simulink model "MdXX_StatusToNetWork"  (R2024b)
settings: Solver=FixedStepDiscrete  StartTime=0.0  StopTime=10.0  FixedStep=0.01  RelTol=1e-3
undefined symbols (not defined in the file or in its folder): KeSMSbSRSPosNumConfig_Val
(part 1 of 2)
settings Model: Creator=sn2xws  LastModifiedBy=sn55gm
settings Model: ModifiedHistory=|
  | 24.8.20 V3.0.0 557新增Md53 Md56
  | 24.10.15 V3.0.1 新增Md57 58
  | 25.7.4 V3.13.0 新增Md61 Md62
settings SolverCC: AlgebraicLoopSolver=TrustRegion
settings DataIOCC: SaveFormat=StructureWithTime  ReturnWorkspaceOutputs=off
settings OptimizationCC: DefaultParameterBehavior=Inlined  EnhancedBackFolding=on  PassReuseOutputArgsAs=Individual arguments  ZeroExternalMemoryAtStartup=off  ZeroInternalMemoryAtStartup=off  OptimizeBlockOrder=speed  DifferentSizesBufferReuse=on  OptimizationCustomize=off  EfficientTunableParamExpr=on
settings DebuggingCC: ParameterTunabilityLossMsg=error  UnconnectedInputMsg=warning  UnconnectedOutputMsg=warning  UnconnectedLineMsg=warning  ArithmeticOperatorsInVariantConditions=warning
settings ModelReferenceCC: EnableRefExpFcnMdlSchedulingChecks=on  ModelReferenceNumInstancesAllowed=Single
settings SFSimCC: MATLABDynamicMemAlloc=off  CustomCodeUndefinedFunction=UseInterfaceOnly
settings RTWCC: Description=AUTOSAR  SystemTargetFile=autosar.tlc  GenCodeOnly=on  TemplateMakefile=ert_default_tmf  GenerateReport=on  IncludeHyperlinkInReport=on  LaunchReport=on  DataTypeReplacement=CDataTypesFixedWidth  GenerateTraceInfo=on  GenerateTraceReport=on  GenerateTraceReportSl=on  GenerateTraceReportSf=on  GenerateTraceReportEml=on  GenerateCodeMetricsReport=on  GPUComputeCapability=3.5
settings CodeAppCC: ForceParamTrailComments=on  IgnoreCustomStorageClasses=off  OperatorAnnotations=on  SimulinkDataObjDesc=on  SFDataObjDesc=on  InsertBlockDesc=on
settings STFCustomTargetCC: TargetLangStandard=C99 (ISO)  MultiwordLength=256  ParMdlRefBuildCompliant=on  CompOptLevelCompliant=on  IncludeMdlTerminateFcn=off  CombineOutputUpdateFcns=on  SuppressErrorStatus=on  ERTCustomFileBanners=on  SupportNonFinite=off  SupportComplex=off  SupportContinuousTime=off  SupportNonInlinedSFcns=off  RemoveResetFunc=on  MATLABClassNameForMDSCustomization=Simulink.SoftwareTarget.ERTCustomization  AutosarCompliant=on  UseToolchainInfoCompliant=on  LookupTableObjectStructAxisOrder=2,1,3,4,...  LUTObjectStructOrderEvenSpacing=Size,Table,Breakpoints  SystemTargetFile=autosar.tlc
settings ERTTargetCC: TargetLangStandard=C99 (ISO)  ConcurrentExecutionCompliant=off  IncludeMdlTerminateFcn=off  SuppressErrorStatus=on  SupportNonFinite=off  SupportComplex=off  ModelStepFunctionPrototypeControlCompliant=off  CPPClassGenCompliant=off  AutosarCompliant=on  LookupTableObjectStructAxisOrder=2,1,3,4,...  LUTObjectStructOrderEvenSpacing=Size,Table,Breakpoints  ERTCustomFileTemplate=example_file_process.tlc  ERTFilePackagingFormat=Compact  BooleanTrueId=TRUE  BooleanFalseId=FALSE  DynamicArrayContainerType=coder::array

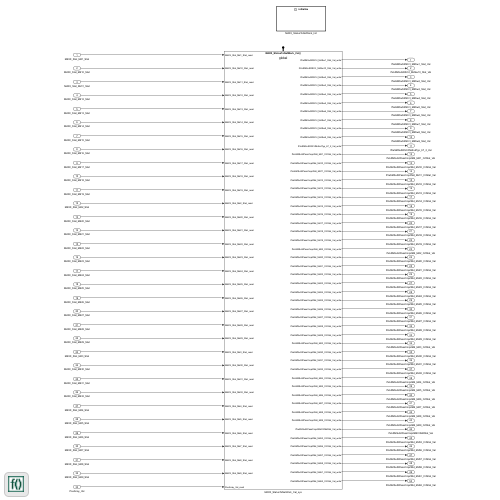
[thumbnail: Simulink's stored preview of the top-level diagram]
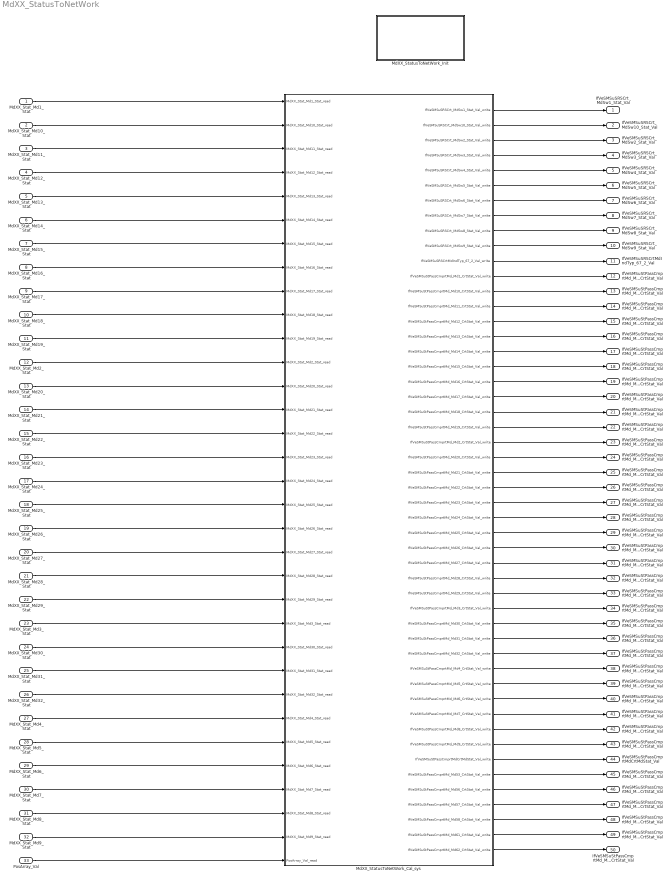
== system MdXX_StatusToNetWork ==
  MdXX_Stat_Md1_Stat : Inport  OutDataTypeStr=uint8  PortDimensions=1
  MdXX_Stat_Md10_Stat : Inport  Port=2  OutDataTypeStr=uint8  PortDimensions=1
  MdXX_Stat_Md11_Stat : Inport  Port=3  OutDataTypeStr=uint8  PortDimensions=1
  MdXX_Stat_Md12_Stat : Inport  Port=4  OutDataTypeStr=uint8  PortDimensions=1
  MdXX_Stat_Md13_Stat : Inport  Port=5  OutDataTypeStr=uint8  PortDimensions=1
  MdXX_Stat_Md14_Stat : Inport  Port=6  OutDataTypeStr=uint8  PortDimensions=1
  MdXX_Stat_Md15_Stat : Inport  Port=7  OutDataTypeStr=uint8  PortDimensions=1
  MdXX_Stat_Md16_Stat : Inport  Port=8  OutDataTypeStr=uint8  PortDimensions=1
  MdXX_Stat_Md17_Stat : Inport  Port=9  OutDataTypeStr=uint8  PortDimensions=1
  MdXX_Stat_Md18_Stat : Inport  Port=10  OutDataTypeStr=uint8  PortDimensions=1
  MdXX_Stat_Md19_Stat : Inport  Port=11  OutDataTypeStr=uint8  PortDimensions=1
  MdXX_Stat_Md2_Stat : Inport  Port=12  OutDataTypeStr=uint8  PortDimensions=1
  MdXX_Stat_Md20_Stat : Inport  Port=13  OutDataTypeStr=uint8  PortDimensions=1
  MdXX_Stat_Md21_Stat : Inport  Port=14  OutDataTypeStr=uint8  PortDimensions=1
  MdXX_Stat_Md22_Stat : Inport  Port=15  OutDataTypeStr=uint8  PortDimensions=1
  MdXX_Stat_Md23_Stat : Inport  Port=16  OutDataTypeStr=uint8  PortDimensions=1
  MdXX_Stat_Md24_Stat : Inport  Port=17  OutDataTypeStr=uint8  PortDimensions=1
  MdXX_Stat_Md25_Stat : Inport  Port=18  OutDataTypeStr=uint8  PortDimensions=1
  MdXX_Stat_Md26_Stat : Inport  Port=19  OutDataTypeStr=uint8  PortDimensions=1
  MdXX_Stat_Md27_Stat : Inport  Port=20  OutDataTypeStr=uint8  PortDimensions=1
  MdXX_Stat_Md28_Stat : Inport  Port=21  OutDataTypeStr=uint8  PortDimensions=1
  MdXX_Stat_Md29_Stat : Inport  Port=22  OutDataTypeStr=uint8  PortDimensions=1
  MdXX_Stat_Md3_Stat : Inport  Port=23  OutDataTypeStr=uint8  PortDimensions=1
  MdXX_Stat_Md30_Stat : Inport  Port=24  OutDataTypeStr=uint8  PortDimensions=1
  MdXX_Stat_Md31_Stat : Inport  Port=25  OutDataTypeStr=uint8  PortDimensions=1
  MdXX_Stat_Md32_Stat : Inport  Port=26  OutDataTypeStr=uint8  PortDimensions=1
  MdXX_Stat_Md4_Stat : Inport  Port=27  OutDataTypeStr=uint8  PortDimensions=1
  MdXX_Stat_Md5_Stat : Inport  Port=28  OutDataTypeStr=uint8  PortDimensions=1
  MdXX_Stat_Md6_Stat : Inport  Port=29  OutDataTypeStr=uint8  PortDimensions=1
  MdXX_Stat_Md7_Stat : Inport  Port=30  OutDataTypeStr=uint8  PortDimensions=1
  MdXX_Stat_Md8_Stat : Inport  Port=31  OutDataTypeStr=uint8  PortDimensions=1
  MdXX_Stat_Md9_Stat : Inport  Port=32  OutDataTypeStr=uint8  PortDimensions=1
  PosArray_Val : Inport  Port=33  OutDataTypeStr=uint8  PortDimensions=11
  MdXX_StatusToNetWork_Cal_sys : Subsystem
  MdXX_StatusToNetWork_Init : Subsystem
  IfVeSMSuSRSCrt_MdSw1_Stat_Val : Outport  OutDataTypeStr=uint8  PortDimensions=1  VectorParamsAs1DForOutWhenUnconnected=off
  IfVeSMSuSRSCrt_MdSw10_Stat_Val : Outport  Port=2  OutDataTypeStr=uint8  PortDimensions=1  VectorParamsAs1DForOutWhenUnconnected=off
  IfVeSMSuSRSCrt_MdSw2_Stat_Val : Outport  Port=3  OutDataTypeStr=uint8  PortDimensions=1  VectorParamsAs1DForOutWhenUnconnected=off
  IfVeSMSuSRSCrt_MdSw3_Stat_Val : Outport  Port=4  OutDataTypeStr=uint8  PortDimensions=1  VectorParamsAs1DForOutWhenUnconnected=off
  IfVeSMSuSRSCrt_MdSw4_Stat_Val : Outport  Port=5  OutDataTypeStr=uint8  PortDimensions=1  VectorParamsAs1DForOutWhenUnconnected=off
  IfVeSMSuSRSCrt_MdSw5_Stat_Val : Outport  Port=6  OutDataTypeStr=uint8  PortDimensions=1  VectorParamsAs1DForOutWhenUnconnected=off
  IfVeSMSuSRSCrt_MdSw6_Stat_Val : Outport  Port=7  OutDataTypeStr=uint8  PortDimensions=1  VectorParamsAs1DForOutWhenUnconnected=off
  IfVeSMSuSRSCrt_MdSw7_Stat_Val : Outport  Port=8  OutDataTypeStr=uint8  PortDimensions=1  VectorParamsAs1DForOutWhenUnconnected=off
  IfVeSMSuSRSCrt_MdSw8_Stat_Val : Outport  Port=9  OutDataTypeStr=uint8  PortDimensions=1  VectorParamsAs1DForOutWhenUnconnected=off
  IfVeSMSuSRSCrt_MdSw9_Stat_Val : Outport  Port=10  OutDataTypeStr=uint8  PortDimensions=1  VectorParamsAs1DForOutWhenUnconnected=off
  IfVeSMSuSRSCrtMdIndTyp_67_2_Val : Outport  Port=11  OutDataTypeStr=uint8  PortDimensions=1  VectorParamsAs1DForOutWhenUnconnected=off
  IfVeSMSuStPassCmprtMd_Md1_CrtStat_Val : Outport  Port=12  OutDataTypeStr=uint8  PortDimensions=1  VectorParamsAs1DForOutWhenUnconnected=off
  IfVeSMSuStPassCmprtMd_Md10_CrtStat_Val : Outport  Port=13  OutDataTypeStr=uint8  PortDimensions=1  VectorParamsAs1DForOutWhenUnconnected=off
  IfVeSMSuStPassCmprtMd_Md11_CrtStat_Val : Outport  Port=14  OutDataTypeStr=uint8  PortDimensions=1  VectorParamsAs1DForOutWhenUnconnected=off
  IfVeSMSuStPassCmprtMd_Md12_CrtStat_Val : Outport  Port=15  OutDataTypeStr=uint8  PortDimensions=1  VectorParamsAs1DForOutWhenUnconnected=off
  IfVeSMSuStPassCmprtMd_Md13_CrtStat_Val : Outport  Port=16  OutDataTypeStr=uint8  PortDimensions=1  VectorParamsAs1DForOutWhenUnconnected=off
  IfVeSMSuStPassCmprtMd_Md14_CrtStat_Val : Outport  Port=17  OutDataTypeStr=uint8  PortDimensions=1  VectorParamsAs1DForOutWhenUnconnected=off
  IfVeSMSuStPassCmprtMd_Md15_CrtStat_Val : Outport  Port=18  OutDataTypeStr=uint8  PortDimensions=1  VectorParamsAs1DForOutWhenUnconnected=off
  IfVeSMSuStPassCmprtMd_Md16_CrtStat_Val : Outport  Port=19  OutDataTypeStr=uint8  PortDimensions=1  VectorParamsAs1DForOutWhenUnconnected=off
  IfVeSMSuStPassCmprtMd_Md17_CrtStat_Val : Outport  Port=20  OutDataTypeStr=uint8  PortDimensions=1  VectorParamsAs1DForOutWhenUnconnected=off
  IfVeSMSuStPassCmprtMd_Md18_CrtStat_Val : Outport  Port=21  OutDataTypeStr=uint8  PortDimensions=1  VectorParamsAs1DForOutWhenUnconnected=off
  IfVeSMSuStPassCmprtMd_Md19_CrtStat_Val : Outport  Port=22  OutDataTypeStr=uint8  PortDimensions=1  VectorParamsAs1DForOutWhenUnconnected=off
  IfVeSMSuStPassCmprtMd_Md2_CrtStat_Val : Outport  Port=23  OutDataTypeStr=uint8  PortDimensions=1  VectorParamsAs1DForOutWhenUnconnected=off
  IfVeSMSuStPassCmprtMd_Md20_CrtStat_Val : Outport  Port=24  OutDataTypeStr=uint8  PortDimensions=1  VectorParamsAs1DForOutWhenUnconnected=off
  IfVeSMSuStPassCmprtMd_Md21_CrtStat_Val : Outport  Port=25  OutDataTypeStr=uint8  PortDimensions=1  VectorParamsAs1DForOutWhenUnconnected=off
  IfVeSMSuStPassCmprtMd_Md22_CrtStat_Val : Outport  Port=26  OutDataTypeStr=uint8  PortDimensions=1  VectorParamsAs1DForOutWhenUnconnected=off
  IfVeSMSuStPassCmprtMd_Md23_CrtStat_Val : Outport  Port=27  OutDataTypeStr=uint8  PortDimensions=1  VectorParamsAs1DForOutWhenUnconnected=off
  IfVeSMSuStPassCmprtMd_Md24_CrtStat_Val : Outport  Port=28  OutDataTypeStr=uint8  PortDimensions=1  VectorParamsAs1DForOutWhenUnconnected=off
  IfVeSMSuStPassCmprtMd_Md25_CrtStat_Val : Outport  Port=29  OutDataTypeStr=uint8  PortDimensions=1  VectorParamsAs1DForOutWhenUnconnected=off
  IfVeSMSuStPassCmprtMd_Md26_CrtStat_Val : Outport  Port=30  OutDataTypeStr=uint8  PortDimensions=1  VectorParamsAs1DForOutWhenUnconnected=off
  IfVeSMSuStPassCmprtMd_Md27_CrtStat_Val : Outport  Port=31  OutDataTypeStr=uint8  PortDimensions=1  VectorParamsAs1DForOutWhenUnconnected=off
  IfVeSMSuStPassCmprtMd_Md28_CrtStat_Val : Outport  Port=32  OutDataTypeStr=uint8  PortDimensions=1  VectorParamsAs1DForOutWhenUnconnected=off
  IfVeSMSuStPassCmprtMd_Md29_CrtStat_Val : Outport  Port=33  OutDataTypeStr=uint8  PortDimensions=1  VectorParamsAs1DForOutWhenUnconnected=off
  IfVeSMSuStPassCmprtMd_Md3_CrtStat_Val : Outport  Port=34  OutDataTypeStr=uint8  PortDimensions=1  VectorParamsAs1DForOutWhenUnconnected=off
  IfVeSMSuStPassCmprtMd_Md30_CrtStat_Val : Outport  Port=35  OutDataTypeStr=uint8  PortDimensions=1  VectorParamsAs1DForOutWhenUnconnected=off
  IfVeSMSuStPassCmprtMd_Md31_CrtStat_Val : Outport  Port=36  OutDataTypeStr=uint8  PortDimensions=1  VectorParamsAs1DForOutWhenUnconnected=off
  IfVeSMSuStPassCmprtMd_Md32_CrtStat_Val : Outport  Port=37  OutDataTypeStr=uint8  PortDimensions=1  VectorParamsAs1DForOutWhenUnconnected=off
  IfVeSMSuStPassCmprtMd_Md4_CrtStat_Val : Outport  Port=38  OutDataTypeStr=uint8  PortDimensions=1  VectorParamsAs1DForOutWhenUnconnected=off
  IfVeSMSuStPassCmprtMd_Md5_CrtStat_Val : Outport  Port=39  OutDataTypeStr=uint8  PortDimensions=1  VectorParamsAs1DForOutWhenUnconnected=off
  IfVeSMSuStPassCmprtMd_Md6_CrtStat_Val : Outport  Port=40  OutDataTypeStr=uint8  PortDimensions=1  VectorParamsAs1DForOutWhenUnconnected=off
  IfVeSMSuStPassCmprtMd_Md7_CrtStat_Val : Outport  Port=41  OutDataTypeStr=uint8  PortDimensions=1  VectorParamsAs1DForOutWhenUnconnected=off
  IfVeSMSuStPassCmprtMd_Md8_CrtStat_Val : Outport  Port=42  OutDataTypeStr=uint8  PortDimensions=1  VectorParamsAs1DForOutWhenUnconnected=off
  IfVeSMSuStPassCmprtMd_Md9_CrtStat_Val : Outport  Port=43  OutDataTypeStr=uint8  PortDimensions=1  VectorParamsAs1DForOutWhenUnconnected=off
  IfVeSMSuStPassCmprtMdCrtMdStat_Val : Outport  Port=44  OutDataTypeStr=uint8  PortDimensions=1  VectorParamsAs1DForOutWhenUnconnected=off
  IfVeSMSuStPassCmprtMd_Md53_CrtStat_Val : Outport  Port=45  OutDataTypeStr=uint8  PortDimensions=1  VectorParamsAs1DForOutWhenUnconnected=off
  IfVeSMSuStPassCmprtMd_Md56_CrtStat_Val : Outport  Port=46  OutDataTypeStr=uint8  PortDimensions=1  VectorParamsAs1DForOutWhenUnconnected=off
  IfVeSMSuStPassCmprtMd_Md57_CrtStat_Val : Outport  Port=47  OutDataTypeStr=uint8  PortDimensions=1  VectorParamsAs1DForOutWhenUnconnected=off
  IfVeSMSuStPassCmprtMd_Md58_CrtStat_Val : Outport  Port=48  OutDataTypeStr=uint8  PortDimensions=1  VectorParamsAs1DForOutWhenUnconnected=off
  IfVeSMSuStPassCmprtMd_Md61_CrtStat_Val : Outport  Port=49  OutDataTypeStr=uint8  PortDimensions=1  VectorParamsAs1DForOutWhenUnconnected=off
  IfVeSMSuStPassCmprtMd_Md62_CrtStat_Val : Outport  Port=50  OutDataTypeStr=uint8  PortDimensions=1  VectorParamsAs1DForOutWhenUnconnected=off
  wires:
  MdXX_Stat_Md1_Stat/1 -> MdXX_StatusToNetWork_Cal_sys/1(MdXX_Stat_Md1_Stat_read)
  MdXX_Stat_Md10_Stat/1 -> MdXX_StatusToNetWork_Cal_sys/2(MdXX_Stat_Md10_Stat_read)
  MdXX_Stat_Md11_Stat/1 -> MdXX_StatusToNetWork_Cal_sys/3(MdXX_Stat_Md11_Stat_read)
  MdXX_Stat_Md12_Stat/1 -> MdXX_StatusToNetWork_Cal_sys/4(MdXX_Stat_Md12_Stat_read)
  MdXX_Stat_Md13_Stat/1 -> MdXX_StatusToNetWork_Cal_sys/5(MdXX_Stat_Md13_Stat_read)
  MdXX_Stat_Md14_Stat/1 -> MdXX_StatusToNetWork_Cal_sys/6(MdXX_Stat_Md14_Stat_read)
  MdXX_Stat_Md15_Stat/1 -> MdXX_StatusToNetWork_Cal_sys/7(MdXX_Stat_Md15_Stat_read)
  MdXX_Stat_Md16_Stat/1 -> MdXX_StatusToNetWork_Cal_sys/8(MdXX_Stat_Md16_Stat_read)
  MdXX_Stat_Md17_Stat/1 -> MdXX_StatusToNetWork_Cal_sys/9(MdXX_Stat_Md17_Stat_read)
  MdXX_Stat_Md18_Stat/1 -> MdXX_StatusToNetWork_Cal_sys/10(MdXX_Stat_Md18_Stat_read)
  MdXX_Stat_Md19_Stat/1 -> MdXX_StatusToNetWork_Cal_sys/11(MdXX_Stat_Md19_Stat_read)
  MdXX_Stat_Md2_Stat/1 -> MdXX_StatusToNetWork_Cal_sys/12(MdXX_Stat_Md2_Stat_read)
  MdXX_Stat_Md20_Stat/1 -> MdXX_StatusToNetWork_Cal_sys/13(MdXX_Stat_Md20_Stat_read)
  MdXX_Stat_Md21_Stat/1 -> MdXX_StatusToNetWork_Cal_sys/14(MdXX_Stat_Md21_Stat_read)
  MdXX_Stat_Md22_Stat/1 -> MdXX_StatusToNetWork_Cal_sys/15(MdXX_Stat_Md22_Stat_read)
  MdXX_Stat_Md23_Stat/1 -> MdXX_StatusToNetWork_Cal_sys/16(MdXX_Stat_Md23_Stat_read)
  MdXX_Stat_Md24_Stat/1 -> MdXX_StatusToNetWork_Cal_sys/17(MdXX_Stat_Md24_Stat_read)
  MdXX_Stat_Md25_Stat/1 -> MdXX_StatusToNetWork_Cal_sys/18(MdXX_Stat_Md25_Stat_read)
  MdXX_Stat_Md26_Stat/1 -> MdXX_StatusToNetWork_Cal_sys/19(MdXX_Stat_Md26_Stat_read)
  MdXX_Stat_Md27_Stat/1 -> MdXX_StatusToNetWork_Cal_sys/20(MdXX_Stat_Md27_Stat_read)
  MdXX_Stat_Md28_Stat/1 -> MdXX_StatusToNetWork_Cal_sys/21(MdXX_Stat_Md28_Stat_read)
  MdXX_Stat_Md29_Stat/1 -> MdXX_StatusToNetWork_Cal_sys/22(MdXX_Stat_Md29_Stat_read)
  MdXX_Stat_Md3_Stat/1 -> MdXX_StatusToNetWork_Cal_sys/23(MdXX_Stat_Md3_Stat_read)
  MdXX_Stat_Md30_Stat/1 -> MdXX_StatusToNetWork_Cal_sys/24(MdXX_Stat_Md30_Stat_read)
  MdXX_Stat_Md31_Stat/1 -> MdXX_StatusToNetWork_Cal_sys/25(MdXX_Stat_Md31_Stat_read)
  MdXX_Stat_Md32_Stat/1 -> MdXX_StatusToNetWork_Cal_sys/26(MdXX_Stat_Md32_Stat_read)
  MdXX_Stat_Md4_Stat/1 -> MdXX_StatusToNetWork_Cal_sys/27(MdXX_Stat_Md4_Stat_read)
  MdXX_Stat_Md5_Stat/1 -> MdXX_StatusToNetWork_Cal_sys/28(MdXX_Stat_Md5_Stat_read)
  MdXX_Stat_Md6_Stat/1 -> MdXX_StatusToNetWork_Cal_sys/29(MdXX_Stat_Md6_Stat_read)
  MdXX_Stat_Md7_Stat/1 -> MdXX_StatusToNetWork_Cal_sys/30(MdXX_Stat_Md7_Stat_read)
  MdXX_Stat_Md8_Stat/1 -> MdXX_StatusToNetWork_Cal_sys/31(MdXX_Stat_Md8_Stat_read)
  MdXX_Stat_Md9_Stat/1 -> MdXX_StatusToNetWork_Cal_sys/32(MdXX_Stat_Md9_Stat_read)
  PosArray_Val/1 -> MdXX_StatusToNetWork_Cal_sys/33(PosArray_Val_read)
  MdXX_StatusToNetWork_Cal_sys/1(IfVeSMSuSRSCrt_MdSw1_Stat_Val_write) -> IfVeSMSuSRSCrt_MdSw1_Stat_Val/1
  MdXX_StatusToNetWork_Cal_sys/2(IfVeSMSuSRSCrt_MdSw10_Stat_Val_write) -> IfVeSMSuSRSCrt_MdSw10_Stat_Val/1
  MdXX_StatusToNetWork_Cal_sys/3(IfVeSMSuSRSCrt_MdSw2_Stat_Val_write) -> IfVeSMSuSRSCrt_MdSw2_Stat_Val/1
  MdXX_StatusToNetWork_Cal_sys/4(IfVeSMSuSRSCrt_MdSw3_Stat_Val_write) -> IfVeSMSuSRSCrt_MdSw3_Stat_Val/1
  MdXX_StatusToNetWork_Cal_sys/5(IfVeSMSuSRSCrt_MdSw4_Stat_Val_write) -> IfVeSMSuSRSCrt_MdSw4_Stat_Val/1
  MdXX_StatusToNetWork_Cal_sys/6(IfVeSMSuSRSCrt_MdSw5_Stat_Val_write) -> IfVeSMSuSRSCrt_MdSw5_Stat_Val/1
  MdXX_StatusToNetWork_Cal_sys/7(IfVeSMSuSRSCrt_MdSw6_Stat_Val_write) -> IfVeSMSuSRSCrt_MdSw6_Stat_Val/1
  MdXX_StatusToNetWork_Cal_sys/8(IfVeSMSuSRSCrt_MdSw7_Stat_Val_write) -> IfVeSMSuSRSCrt_MdSw7_Stat_Val/1
  MdXX_StatusToNetWork_Cal_sys/9(IfVeSMSuSRSCrt_MdSw8_Stat_Val_write) -> IfVeSMSuSRSCrt_MdSw8_Stat_Val/1
  MdXX_StatusToNetWork_Cal_sys/10(IfVeSMSuSRSCrt_MdSw9_Stat_Val_write) -> IfVeSMSuSRSCrt_MdSw9_Stat_Val/1
  MdXX_StatusToNetWork_Cal_sys/11(IfVeSMSuSRSCrtMdIndTyp_67_2_Val_write) -> IfVeSMSuSRSCrtMdIndTyp_67_2_Val/1
  MdXX_StatusToNetWork_Cal_sys/12(IfVeSMSuStPassCmprtMd_Md1_CrtStat_Val_write) -> IfVeSMSuStPassCmprtMd_Md1_CrtStat_Val/1
  MdXX_StatusToNetWork_Cal_sys/13(IfVeSMSuStPassCmprtMd_Md10_CrtStat_Val_write) -> IfVeSMSuStPassCmprtMd_Md10_CrtStat_Val/1
  MdXX_StatusToNetWork_Cal_sys/14(IfVeSMSuStPassCmprtMd_Md11_CrtStat_Val_write) -> IfVeSMSuStPassCmprtMd_Md11_CrtStat_Val/1
  MdXX_StatusToNetWork_Cal_sys/15(IfVeSMSuStPassCmprtMd_Md12_CrtStat_Val_write) -> IfVeSMSuStPassCmprtMd_Md12_CrtStat_Val/1
  MdXX_StatusToNetWork_Cal_sys/16(IfVeSMSuStPassCmprtMd_Md13_CrtStat_Val_write) -> IfVeSMSuStPassCmprtMd_Md13_CrtStat_Val/1
  MdXX_StatusToNetWork_Cal_sys/17(IfVeSMSuStPassCmprtMd_Md14_CrtStat_Val_write) -> IfVeSMSuStPassCmprtMd_Md14_CrtStat_Val/1
  MdXX_StatusToNetWork_Cal_sys/18(IfVeSMSuStPassCmprtMd_Md15_CrtStat_Val_write) -> IfVeSMSuStPassCmprtMd_Md15_CrtStat_Val/1
  MdXX_StatusToNetWork_Cal_sys/19(IfVeSMSuStPassCmprtMd_Md16_CrtStat_Val_write) -> IfVeSMSuStPassCmprtMd_Md16_CrtStat_Val/1
  MdXX_StatusToNetWork_Cal_sys/20(IfVeSMSuStPassCmprtMd_Md17_CrtStat_Val_write) -> IfVeSMSuStPassCmprtMd_Md17_CrtStat_Val/1
  MdXX_StatusToNetWork_Cal_sys/21(IfVeSMSuStPassCmprtMd_Md18_CrtStat_Val_write) -> IfVeSMSuStPassCmprtMd_Md18_CrtStat_Val/1
  MdXX_StatusToNetWork_Cal_sys/22(IfVeSMSuStPassCmprtMd_Md19_CrtStat_Val_write) -> IfVeSMSuStPassCmprtMd_Md19_CrtStat_Val/1
  MdXX_StatusToNetWork_Cal_sys/23(IfVeSMSuStPassCmprtMd_Md2_CrtStat_Val_write) -> IfVeSMSuStPassCmprtMd_Md2_CrtStat_Val/1
  MdXX_StatusToNetWork_Cal_sys/24(IfVeSMSuStPassCmprtMd_Md20_CrtStat_Val_write) -> IfVeSMSuStPassCmprtMd_Md20_CrtStat_Val/1
  MdXX_StatusToNetWork_Cal_sys/25(IfVeSMSuStPassCmprtMd_Md21_CrtStat_Val_write) -> IfVeSMSuStPassCmprtMd_Md21_CrtStat_Val/1
  MdXX_StatusToNetWork_Cal_sys/26(IfVeSMSuStPassCmprtMd_Md22_CrtStat_Val_write) -> IfVeSMSuStPassCmprtMd_Md22_CrtStat_Val/1
  MdXX_StatusToNetWork_Cal_sys/27(IfVeSMSuStPassCmprtMd_Md23_CrtStat_Val_write) -> IfVeSMSuStPassCmprtMd_Md23_CrtStat_Val/1
  MdXX_StatusToNetWork_Cal_sys/28(IfVeSMSuStPassCmprtMd_Md24_CrtStat_Val_write) -> IfVeSMSuStPassCmprtMd_Md24_CrtStat_Val/1
  MdXX_StatusToNetWork_Cal_sys/29(IfVeSMSuStPassCmprtMd_Md25_CrtStat_Val_write) -> IfVeSMSuStPassCmprtMd_Md25_CrtStat_Val/1
  MdXX_StatusToNetWork_Cal_sys/30(IfVeSMSuStPassCmprtMd_Md26_CrtStat_Val_write) -> IfVeSMSuStPassCmprtMd_Md26_CrtStat_Val/1
  MdXX_StatusToNetWork_Cal_sys/31(IfVeSMSuStPassCmprtMd_Md27_CrtStat_Val_write) -> IfVeSMSuStPassCmprtMd_Md27_CrtStat_Val/1
  MdXX_StatusToNetWork_Cal_sys/32(IfVeSMSuStPassCmprtMd_Md28_CrtStat_Val_write) -> IfVeSMSuStPassCmprtMd_Md28_CrtStat_Val/1
  MdXX_StatusToNetWork_Cal_sys/33(IfVeSMSuStPassCmprtMd_Md29_CrtStat_Val_write) -> IfVeSMSuStPassCmprtMd_Md29_CrtStat_Val/1
  MdXX_StatusToNetWork_Cal_sys/34(IfVeSMSuStPassCmprtMd_Md3_CrtStat_Val_write) -> IfVeSMSuStPassCmprtMd_Md3_CrtStat_Val/1
  MdXX_StatusToNetWork_Cal_sys/35(IfVeSMSuStPassCmprtMd_Md30_CrtStat_Val_write) -> IfVeSMSuStPassCmprtMd_Md30_CrtStat_Val/1
  MdXX_StatusToNetWork_Cal_sys/36(IfVeSMSuStPassCmprtMd_Md31_CrtStat_Val_write) -> IfVeSMSuStPassCmprtMd_Md31_CrtStat_Val/1
  MdXX_StatusToNetWork_Cal_sys/37(IfVeSMSuStPassCmprtMd_Md32_CrtStat_Val_write) -> IfVeSMSuStPassCmprtMd_Md32_CrtStat_Val/1
  MdXX_StatusToNetWork_Cal_sys/38(IfVeSMSuStPassCmprtMd_Md4_CrtStat_Val_write) -> IfVeSMSuStPassCmprtMd_Md4_CrtStat_Val/1
  MdXX_StatusToNetWork_Cal_sys/39(IfVeSMSuStPassCmprtMd_Md5_CrtStat_Val_write) -> IfVeSMSuStPassCmprtMd_Md5_CrtStat_Val/1
  MdXX_StatusToNetWork_Cal_sys/40(IfVeSMSuStPassCmprtMd_Md6_CrtStat_Val_write) -> IfVeSMSuStPassCmprtMd_Md6_CrtStat_Val/1
  MdXX_StatusToNetWork_Cal_sys/41(IfVeSMSuStPassCmprtMd_Md7_CrtStat_Val_write) -> IfVeSMSuStPassCmprtMd_Md7_CrtStat_Val/1
  MdXX_StatusToNetWork_Cal_sys/42(IfVeSMSuStPassCmprtMd_Md8_CrtStat_Val_write) -> IfVeSMSuStPassCmprtMd_Md8_CrtStat_Val/1
  MdXX_StatusToNetWork_Cal_sys/43(IfVeSMSuStPassCmprtMd_Md9_CrtStat_Val_write) -> IfVeSMSuStPassCmprtMd_Md9_CrtStat_Val/1
  MdXX_StatusToNetWork_Cal_sys/44(IfVeSMSuStPassCmprtMdCrtMdStat_Val_write) -> IfVeSMSuStPassCmprtMdCrtMdStat_Val/1
  MdXX_StatusToNetWork_Cal_sys/45(IfVeSMSuStPassCmprtMd_Md53_CrtStat_Val_write) -> IfVeSMSuStPassCmprtMd_Md53_CrtStat_Val/1
  MdXX_StatusToNetWork_Cal_sys/46(IfVeSMSuStPassCmprtMd_Md56_CrtStat_Val_write) -> IfVeSMSuStPassCmprtMd_Md56_CrtStat_Val/1
  MdXX_StatusToNetWork_Cal_sys/47(IfVeSMSuStPassCmprtMd_Md57_CrtStat_Val_write) -> IfVeSMSuStPassCmprtMd_Md57_CrtStat_Val/1
  MdXX_StatusToNetWork_Cal_sys/48(IfVeSMSuStPassCmprtMd_Md58_CrtStat_Val_write) -> IfVeSMSuStPassCmprtMd_Md58_CrtStat_Val/1
  MdXX_StatusToNetWork_Cal_sys/49(IfVeSMSuStPassCmprtMd_Md61_CrtStat_Val_write) -> IfVeSMSuStPassCmprtMd_Md61_CrtStat_Val/1
  MdXX_StatusToNetWork_Cal_sys/50(IfVeSMSuStPassCmprtMd_Md62_CrtStat_Val_write) -> IfVeSMSuStPassCmprtMd_Md62_CrtStat_Val/1

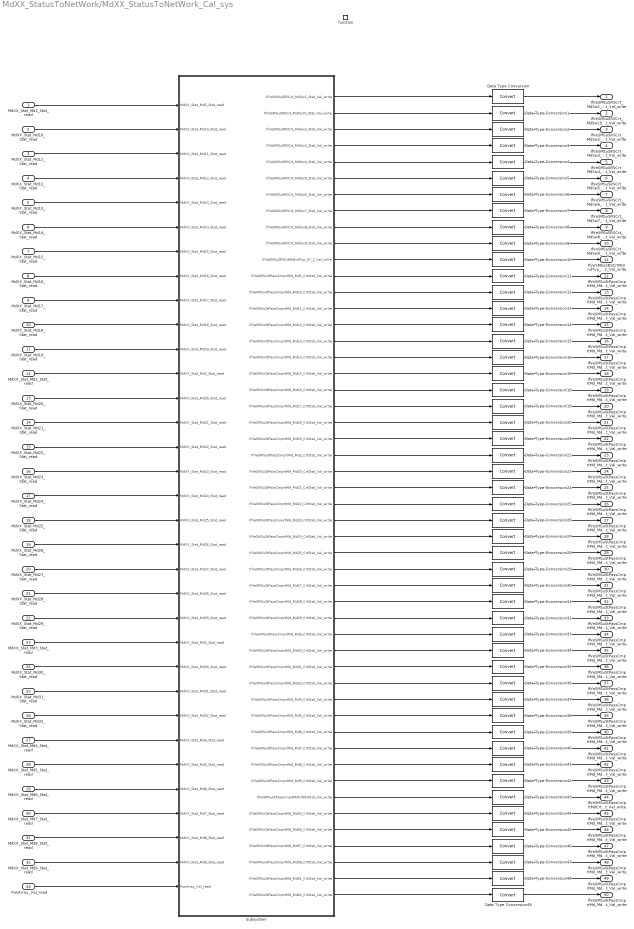
== system MdXX_StatusToNetWork/MdXX_StatusToNetWork_Cal_sys ==
  MdXX_Stat_Md1_Stat_read : Inport
  MdXX_Stat_Md10_Stat_read : Inport  Port=2
  MdXX_Stat_Md11_Stat_read : Inport  Port=3
  MdXX_Stat_Md12_Stat_read : Inport  Port=4
  MdXX_Stat_Md13_Stat_read : Inport  Port=5
  MdXX_Stat_Md14_Stat_read : Inport  Port=6
  MdXX_Stat_Md15_Stat_read : Inport  Port=7
  MdXX_Stat_Md16_Stat_read : Inport  Port=8
  MdXX_Stat_Md17_Stat_read : Inport  Port=9
  MdXX_Stat_Md18_Stat_read : Inport  Port=10
  MdXX_Stat_Md19_Stat_read : Inport  Port=11
  MdXX_Stat_Md2_Stat_read : Inport  Port=12
  MdXX_Stat_Md20_Stat_read : Inport  Port=13
  MdXX_Stat_Md21_Stat_read : Inport  Port=14
  MdXX_Stat_Md22_Stat_read : Inport  Port=15
  MdXX_Stat_Md23_Stat_read : Inport  Port=16
  MdXX_Stat_Md24_Stat_read : Inport  Port=17
  MdXX_Stat_Md25_Stat_read : Inport  Port=18
  MdXX_Stat_Md26_Stat_read : Inport  Port=19
  MdXX_Stat_Md27_Stat_read : Inport  Port=20
  MdXX_Stat_Md28_Stat_read : Inport  Port=21
  MdXX_Stat_Md29_Stat_read : Inport  Port=22
  MdXX_Stat_Md3_Stat_read : Inport  Port=23
  MdXX_Stat_Md30_Stat_read : Inport  Port=24
  MdXX_Stat_Md31_Stat_read : Inport  Port=25
  MdXX_Stat_Md32_Stat_read : Inport  Port=26
  MdXX_Stat_Md4_Stat_read : Inport  Port=27
  MdXX_Stat_Md5_Stat_read : Inport  Port=28
  MdXX_Stat_Md6_Stat_read : Inport  Port=29
  MdXX_Stat_Md7_Stat_read : Inport  Port=30
  MdXX_Stat_Md8_Stat_read : Inport  Port=31
  MdXX_Stat_Md9_Stat_read : Inport  Port=32
  PosArray_Val_read : Inport  Port=33
  function : TriggerPort  TriggerType=function-call  IsSimulinkFunction=on  FunctionName=MdXX_StatusToNetWork_Cal  VariantControl=(inherit)
  Data Type Conversion{,1..49} (50 alike) : DataTypeConversion  SaturateOnIntegerOverflow=off  RndMeth=Floor
  Subsystem : Subsystem
  IfVeSMSuSRSCrt_MdSw1_Stat_Val_write : Outport  VectorParamsAs1DForOutWhenUnconnected=off
      settings: EnsureOutportIsVirtual=on
  IfVeSMSuSRSCrt_MdSw10_Stat_Val_write : Outport  Port=2  VectorParamsAs1DForOutWhenUnconnected=off
      settings: EnsureOutportIsVirtual=on
  IfVeSMSuSRSCrt_MdSw2_Stat_Val_write : Outport  Port=3  VectorParamsAs1DForOutWhenUnconnected=off
      settings: EnsureOutportIsVirtual=on
  IfVeSMSuSRSCrt_MdSw3_Stat_Val_write : Outport  Port=4  VectorParamsAs1DForOutWhenUnconnected=off
      settings: EnsureOutportIsVirtual=on
  IfVeSMSuSRSCrt_MdSw4_Stat_Val_write : Outport  Port=5  VectorParamsAs1DForOutWhenUnconnected=off
      settings: EnsureOutportIsVirtual=on
  IfVeSMSuSRSCrt_MdSw5_Stat_Val_write : Outport  Port=6  VectorParamsAs1DForOutWhenUnconnected=off
      settings: EnsureOutportIsVirtual=on
  IfVeSMSuSRSCrt_MdSw6_Stat_Val_write : Outport  Port=7  VectorParamsAs1DForOutWhenUnconnected=off
      settings: EnsureOutportIsVirtual=on
  IfVeSMSuSRSCrt_MdSw7_Stat_Val_write : Outport  Port=8  VectorParamsAs1DForOutWhenUnconnected=off
      settings: EnsureOutportIsVirtual=on
  IfVeSMSuSRSCrt_MdSw8_Stat_Val_write : Outport  Port=9  VectorParamsAs1DForOutWhenUnconnected=off
      settings: EnsureOutportIsVirtual=on
  IfVeSMSuSRSCrt_MdSw9_Stat_Val_write : Outport  Port=10  VectorParamsAs1DForOutWhenUnconnected=off
      settings: EnsureOutportIsVirtual=on
  IfVeSMSuSRSCrtMdIndTyp_67_2_Val_write : Outport  Port=11  VectorParamsAs1DForOutWhenUnconnected=off
      settings: EnsureOutportIsVirtual=on
  IfVeSMSuStPassCmprtMd_Md1_CrtStat_Val_write : Outport  Port=12  VectorParamsAs1DForOutWhenUnconnected=off
      settings: EnsureOutportIsVirtual=on
  IfVeSMSuStPassCmprtMd_Md10_CrtStat_Val_write : Outport  Port=13  VectorParamsAs1DForOutWhenUnconnected=off
      settings: EnsureOutportIsVirtual=on
  IfVeSMSuStPassCmprtMd_Md11_CrtStat_Val_write : Outport  Port=14  VectorParamsAs1DForOutWhenUnconnected=off
      settings: EnsureOutportIsVirtual=on
  IfVeSMSuStPassCmprtMd_Md12_CrtStat_Val_write : Outport  Port=15  VectorParamsAs1DForOutWhenUnconnected=off
      settings: EnsureOutportIsVirtual=on
  IfVeSMSuStPassCmprtMd_Md13_CrtStat_Val_write : Outport  Port=16  VectorParamsAs1DForOutWhenUnconnected=off
      settings: EnsureOutportIsVirtual=on
  IfVeSMSuStPassCmprtMd_Md14_CrtStat_Val_write : Outport  Port=17  VectorParamsAs1DForOutWhenUnconnected=off
      settings: EnsureOutportIsVirtual=on
  IfVeSMSuStPassCmprtMd_Md15_CrtStat_Val_write : Outport  Port=18  VectorParamsAs1DForOutWhenUnconnected=off
      settings: EnsureOutportIsVirtual=on
  IfVeSMSuStPassCmprtMd_Md16_CrtStat_Val_write : Outport  Port=19  VectorParamsAs1DForOutWhenUnconnected=off
      settings: EnsureOutportIsVirtual=on
  IfVeSMSuStPassCmprtMd_Md17_CrtStat_Val_write : Outport  Port=20  VectorParamsAs1DForOutWhenUnconnected=off
      settings: EnsureOutportIsVirtual=on
  IfVeSMSuStPassCmprtMd_Md18_CrtStat_Val_write : Outport  Port=21  VectorParamsAs1DForOutWhenUnconnected=off
      settings: EnsureOutportIsVirtual=on
  IfVeSMSuStPassCmprtMd_Md19_CrtStat_Val_write : Outport  Port=22  VectorParamsAs1DForOutWhenUnconnected=off
      settings: EnsureOutportIsVirtual=on
  IfVeSMSuStPassCmprtMd_Md2_CrtStat_Val_write : Outport  Port=23  VectorParamsAs1DForOutWhenUnconnected=off
      settings: EnsureOutportIsVirtual=on
  IfVeSMSuStPassCmprtMd_Md20_CrtStat_Val_write : Outport  Port=24  VectorParamsAs1DForOutWhenUnconnected=off
      settings: EnsureOutportIsVirtual=on
  IfVeSMSuStPassCmprtMd_Md21_CrtStat_Val_write : Outport  Port=25  VectorParamsAs1DForOutWhenUnconnected=off
      settings: EnsureOutportIsVirtual=on
  IfVeSMSuStPassCmprtMd_Md22_CrtStat_Val_write : Outport  Port=26  VectorParamsAs1DForOutWhenUnconnected=off
      settings: EnsureOutportIsVirtual=on
  IfVeSMSuStPassCmprtMd_Md23_CrtStat_Val_write : Outport  Port=27  VectorParamsAs1DForOutWhenUnconnected=off
      settings: EnsureOutportIsVirtual=on
  IfVeSMSuStPassCmprtMd_Md24_CrtStat_Val_write : Outport  Port=28  VectorParamsAs1DForOutWhenUnconnected=off
      settings: EnsureOutportIsVirtual=on
  IfVeSMSuStPassCmprtMd_Md25_CrtStat_Val_write : Outport  Port=29  VectorParamsAs1DForOutWhenUnconnected=off
      settings: EnsureOutportIsVirtual=on
  IfVeSMSuStPassCmprtMd_Md26_CrtStat_Val_write : Outport  Port=30  VectorParamsAs1DForOutWhenUnconnected=off
      settings: EnsureOutportIsVirtual=on
  IfVeSMSuStPassCmprtMd_Md27_CrtStat_Val_write : Outport  Port=31  VectorParamsAs1DForOutWhenUnconnected=off
      settings: EnsureOutportIsVirtual=on
  IfVeSMSuStPassCmprtMd_Md28_CrtStat_Val_write : Outport  Port=32  VectorParamsAs1DForOutWhenUnconnected=off
      settings: EnsureOutportIsVirtual=on
  IfVeSMSuStPassCmprtMd_Md29_CrtStat_Val_write : Outport  Port=33  VectorParamsAs1DForOutWhenUnconnected=off
      settings: EnsureOutportIsVirtual=on
  IfVeSMSuStPassCmprtMd_Md3_CrtStat_Val_write : Outport  Port=34  VectorParamsAs1DForOutWhenUnconnected=off
      settings: EnsureOutportIsVirtual=on
  IfVeSMSuStPassCmprtMd_Md30_CrtStat_Val_write : Outport  Port=35  VectorParamsAs1DForOutWhenUnconnected=off
      settings: EnsureOutportIsVirtual=on
  IfVeSMSuStPassCmprtMd_Md31_CrtStat_Val_write : Outport  Port=36  VectorParamsAs1DForOutWhenUnconnected=off
      settings: EnsureOutportIsVirtual=on
  IfVeSMSuStPassCmprtMd_Md32_CrtStat_Val_write : Outport  Port=37  VectorParamsAs1DForOutWhenUnconnected=off
      settings: EnsureOutportIsVirtual=on
  IfVeSMSuStPassCmprtMd_Md4_CrtStat_Val_write : Outport  Port=38  VectorParamsAs1DForOutWhenUnconnected=off
      settings: EnsureOutportIsVirtual=on
  IfVeSMSuStPassCmprtMd_Md5_CrtStat_Val_write : Outport  Port=39  VectorParamsAs1DForOutWhenUnconnected=off
      settings: EnsureOutportIsVirtual=on
  IfVeSMSuStPassCmprtMd_Md6_CrtStat_Val_write : Outport  Port=40  VectorParamsAs1DForOutWhenUnconnected=off
      settings: EnsureOutportIsVirtual=on
  IfVeSMSuStPassCmprtMd_Md7_CrtStat_Val_write : Outport  Port=41  VectorParamsAs1DForOutWhenUnconnected=off
      settings: EnsureOutportIsVirtual=on
  IfVeSMSuStPassCmprtMd_Md8_CrtStat_Val_write : Outport  Port=42  VectorParamsAs1DForOutWhenUnconnected=off
      settings: EnsureOutportIsVirtual=on
  IfVeSMSuStPassCmprtMd_Md9_CrtStat_Val_write : Outport  Port=43  VectorParamsAs1DForOutWhenUnconnected=off
      settings: EnsureOutportIsVirtual=on
  IfVeSMSuStPassCmprtMdCrtMdStat_Val_write : Outport  Port=44  VectorParamsAs1DForOutWhenUnconnected=off
      settings: EnsureOutportIsVirtual=on
  IfVeSMSuStPassCmprtMd_Md53_CrtStat_Val_write : Outport  Port=45  VectorParamsAs1DForOutWhenUnconnected=off
      settings: EnsureOutportIsVirtual=on
  IfVeSMSuStPassCmprtMd_Md56_CrtStat_Val_write : Outport  Port=46  VectorParamsAs1DForOutWhenUnconnected=off
      settings: EnsureOutportIsVirtual=on
  IfVeSMSuStPassCmprtMd_Md57_CrtStat_Val_write : Outport  Port=47  VectorParamsAs1DForOutWhenUnconnected=off
      settings: EnsureOutportIsVirtual=on
  IfVeSMSuStPassCmprtMd_Md58_CrtStat_Val_write : Outport  Port=48  VectorParamsAs1DForOutWhenUnconnected=off
      settings: EnsureOutportIsVirtual=on
  IfVeSMSuStPassCmprtMd_Md61_CrtStat_Val_write : Outport  Port=49  VectorParamsAs1DForOutWhenUnconnected=off
      settings: EnsureOutportIsVirtual=on
  IfVeSMSuStPassCmprtMd_Md62_CrtStat_Val_write : Outport  Port=50  VectorParamsAs1DForOutWhenUnconnected=off
      settings: EnsureOutportIsVirtual=on
  wires:
  Subsystem/43(IfVeSMSuStPassCmprtMd_Md9_CrtStat_Val_write) -> Data Type Conversion42/1
  Subsystem/15(IfVeSMSuStPassCmprtMd_Md12_CrtStat_Val_write) -> Data Type Conversion14/1
  Subsystem/38(IfVeSMSuStPassCmprtMd_Md4_CrtStat_Val_write) -> Data Type Conversion37/1
  Subsystem/44(IfVeSMSuStPassCmprtMdCrtMdStat_Val_write) -> Data Type Conversion43/1
  Subsystem/31(IfVeSMSuStPassCmprtMd_Md27_CrtStat_Val_write) -> Data Type Conversion30/1
  Subsystem/37(IfVeSMSuStPassCmprtMd_Md32_CrtStat_Val_write) -> Data Type Conversion36/1
  Subsystem/34(IfVeSMSuStPassCmprtMd_Md3_CrtStat_Val_write) -> Data Type Conversion33/1
  Subsystem/8(IfVeSMSuSRSCrt_MdSw7_Stat_Val_write) -> Data Type Conversion7/1
  Subsystem/4(IfVeSMSuSRSCrt_MdSw3_Stat_Val_write) -> Data Type Conversion3/1
  Subsystem/35(IfVeSMSuStPassCmprtMd_Md30_CrtStat_Val_write) -> Data Type Conversion34/1
  Subsystem/18(IfVeSMSuStPassCmprtMd_Md15_CrtStat_Val_write) -> Data Type Conversion17/1
  Subsystem/29(IfVeSMSuStPassCmprtMd_Md25_CrtStat_Val_write) -> Data Type Conversion28/1
  Subsystem/24(IfVeSMSuStPassCmprtMd_Md20_CrtStat_Val_write) -> Data Type Conversion23/1
  Subsystem/33(IfVeSMSuStPassCmprtMd_Md29_CrtStat_Val_write) -> Data Type Conversion32/1
  Subsystem/22(IfVeSMSuStPassCmprtMd_Md19_CrtStat_Val_write) -> Data Type Conversion21/1
  Subsystem/32(IfVeSMSuStPassCmprtMd_Md28_CrtStat_Val_write) -> Data Type Conversion31/1
  Subsystem/20(IfVeSMSuStPassCmprtMd_Md17_CrtStat_Val_write) -> Data Type Conversion19/1
  Subsystem/42(IfVeSMSuStPassCmprtMd_Md8_CrtStat_Val_write) -> Data Type Conversion41/1
  Subsystem/3(IfVeSMSuSRSCrt_MdSw2_Stat_Val_write) -> Data Type Conversion2/1
  Subsystem/7(IfVeSMSuSRSCrt_MdSw6_Stat_Val_write) -> Data Type Conversion6/1
  Subsystem/41(IfVeSMSuStPassCmprtMd_Md7_CrtStat_Val_write) -> Data Type Conversion40/1
  Subsystem/28(IfVeSMSuStPassCmprtMd_Md24_CrtStat_Val_write) -> Data Type Conversion27/1
  Subsystem/9(IfVeSMSuSRSCrt_MdSw8_Stat_Val_write) -> Data Type Conversion8/1
  Subsystem/14(IfVeSMSuStPassCmprtMd_Md11_CrtStat_Val_write) -> Data Type Conversion13/1
  Subsystem/19(IfVeSMSuStPassCmprtMd_Md16_CrtStat_Val_write) -> Data Type Conversion18/1
  Subsystem/1(IfVeSMSuSRSCrt_MdSw1_Stat_Val_write) -> Data Type Conversion/1
  Subsystem/36(IfVeSMSuStPassCmprtMd_Md31_CrtStat_Val_write) -> Data Type Conversion35/1
  Subsystem/6(IfVeSMSuSRSCrt_MdSw5_Stat_Val_write) -> Data Type Conversion5/1
  Subsystem/11(IfVeSMSuSRSCrtMdIndTyp_67_2_Val_write) -> Data Type Conversion10/1
  Subsystem/25(IfVeSMSuStPassCmprtMd_Md21_CrtStat_Val_write) -> Data Type Conversion24/1
  Subsystem/30(IfVeSMSuStPassCmprtMd_Md26_CrtStat_Val_write) -> Data Type Conversion29/1
  Subsystem/27(IfVeSMSuStPassCmprtMd_Md23_CrtStat_Val_write) -> Data Type Conversion26/1
  Subsystem/10(IfVeSMSuSRSCrt_MdSw9_Stat_Val_write) -> Data Type Conversion9/1
  Subsystem/23(IfVeSMSuStPassCmprtMd_Md2_CrtStat_Val_write) -> Data Type Conversion22/1
  Subsystem/16(IfVeSMSuStPassCmprtMd_Md13_CrtStat_Val_write) -> Data Type Conversion15/1
  Subsystem/17(IfVeSMSuStPassCmprtMd_Md14_CrtStat_Val_write) -> Data Type Conversion16/1
  Subsystem/40(IfVeSMSuStPassCmprtMd_Md6_CrtStat_Val_write) -> Data Type Conversion39/1
  Subsystem/26(IfVeSMSuStPassCmprtMd_Md22_CrtStat_Val_write) -> Data Type Conversion25/1
  Subsystem/5(IfVeSMSuSRSCrt_MdSw4_Stat_Val_write) -> Data Type Conversion4/1
  Subsystem/13(IfVeSMSuStPassCmprtMd_Md10_CrtStat_Val_write) -> Data Type Conversion12/1
  Subsystem/21(IfVeSMSuStPassCmprtMd_Md18_CrtStat_Val_write) -> Data Type Conversion20/1
  Subsystem/2(IfVeSMSuSRSCrt_MdSw10_Stat_Val_write) -> Data Type Conversion1/1
  Subsystem/39(IfVeSMSuStPassCmprtMd_Md5_CrtStat_Val_write) -> Data Type Conversion38/1
  Subsystem/12(IfVeSMSuStPassCmprtMd_Md1_CrtStat_Val_write) -> Data Type Conversion11/1
  MdXX_Stat_Md1_Stat_read/1 -> Subsystem/1(MdXX_Stat_Md1_Stat_read)
  MdXX_Stat_Md10_Stat_read/1 -> Subsystem/2(MdXX_Stat_Md10_Stat_read)
  MdXX_Stat_Md11_Stat_read/1 -> Subsystem/3(MdXX_Stat_Md11_Stat_read)
  MdXX_Stat_Md12_Stat_read/1 -> Subsystem/4(MdXX_Stat_Md12_Stat_read)
  MdXX_Stat_Md13_Stat_read/1 -> Subsystem/5(MdXX_Stat_Md13_Stat_read)
  MdXX_Stat_Md14_Stat_read/1 -> Subsystem/6(MdXX_Stat_Md14_Stat_read)
  MdXX_Stat_Md15_Stat_read/1 -> Subsystem/7(MdXX_Stat_Md15_Stat_read)
  MdXX_Stat_Md16_Stat_read/1 -> Subsystem/8(MdXX_Stat_Md16_Stat_read)
  MdXX_Stat_Md17_Stat_read/1 -> Subsystem/9(MdXX_Stat_Md17_Stat_read)
  MdXX_Stat_Md18_Stat_read/1 -> Subsystem/10(MdXX_Stat_Md18_Stat_read)
  MdXX_Stat_Md19_Stat_read/1 -> Subsystem/11(MdXX_Stat_Md19_Stat_read)
  MdXX_Stat_Md2_Stat_read/1 -> Subsystem/12(MdXX_Stat_Md2_Stat_read)
  MdXX_Stat_Md20_Stat_read/1 -> Subsystem/13(MdXX_Stat_Md20_Stat_read)
  MdXX_Stat_Md21_Stat_read/1 -> Subsystem/14(MdXX_Stat_Md21_Stat_read)
  MdXX_Stat_Md22_Stat_read/1 -> Subsystem/15(MdXX_Stat_Md22_Stat_read)
  MdXX_Stat_Md23_Stat_read/1 -> Subsystem/16(MdXX_Stat_Md23_Stat_read)
  MdXX_Stat_Md24_Stat_read/1 -> Subsystem/17(MdXX_Stat_Md24_Stat_read)
  MdXX_Stat_Md25_Stat_read/1 -> Subsystem/18(MdXX_Stat_Md25_Stat_read)
  MdXX_Stat_Md26_Stat_read/1 -> Subsystem/19(MdXX_Stat_Md26_Stat_read)
  MdXX_Stat_Md27_Stat_read/1 -> Subsystem/20(MdXX_Stat_Md27_Stat_read)
  MdXX_Stat_Md28_Stat_read/1 -> Subsystem/21(MdXX_Stat_Md28_Stat_read)
  MdXX_Stat_Md29_Stat_read/1 -> Subsystem/22(MdXX_Stat_Md29_Stat_read)
  MdXX_Stat_Md3_Stat_read/1 -> Subsystem/23(MdXX_Stat_Md3_Stat_read)
  MdXX_Stat_Md30_Stat_read/1 -> Subsystem/24(MdXX_Stat_Md30_Stat_read)
  MdXX_Stat_Md31_Stat_read/1 -> Subsystem/25(MdXX_Stat_Md31_Stat_read)
  MdXX_Stat_Md32_Stat_read/1 -> Subsystem/26(MdXX_Stat_Md32_Stat_read)
  MdXX_Stat_Md4_Stat_read/1 -> Subsystem/27(MdXX_Stat_Md4_Stat_read)
  MdXX_Stat_Md5_Stat_read/1 -> Subsystem/28(MdXX_Stat_Md5_Stat_read)
  MdXX_Stat_Md6_Stat_read/1 -> Subsystem/29(MdXX_Stat_Md6_Stat_read)
  MdXX_Stat_Md7_Stat_read/1 -> Subsystem/30(MdXX_Stat_Md7_Stat_read)
  MdXX_Stat_Md8_Stat_read/1 -> Subsystem/31(MdXX_Stat_Md8_Stat_read)
  MdXX_Stat_Md9_Stat_read/1 -> Subsystem/32(MdXX_Stat_Md9_Stat_read)
  PosArray_Val_read/1 -> Subsystem/33(PosArray_Val_read)
  Data Type Conversion/1 -> IfVeSMSuSRSCrt_MdSw1_Stat_Val_write/1
  Data Type Conversion1/1 -> IfVeSMSuSRSCrt_MdSw10_Stat_Val_write/1
  Data Type Conversion2/1 -> IfVeSMSuSRSCrt_MdSw2_Stat_Val_write/1
  Data Type Conversion3/1 -> IfVeSMSuSRSCrt_MdSw3_Stat_Val_write/1
  Data Type Conversion4/1 -> IfVeSMSuSRSCrt_MdSw4_Stat_Val_write/1
  Data Type Conversion5/1 -> IfVeSMSuSRSCrt_MdSw5_Stat_Val_write/1
  Data Type Conversion6/1 -> IfVeSMSuSRSCrt_MdSw6_Stat_Val_write/1
  Data Type Conversion7/1 -> IfVeSMSuSRSCrt_MdSw7_Stat_Val_write/1
  Data Type Conversion8/1 -> IfVeSMSuSRSCrt_MdSw8_Stat_Val_write/1
  Data Type Conversion9/1 -> IfVeSMSuSRSCrt_MdSw9_Stat_Val_write/1
  Data Type Conversion10/1 -> IfVeSMSuSRSCrtMdIndTyp_67_2_Val_write/1
  Data Type Conversion11/1 -> IfVeSMSuStPassCmprtMd_Md1_CrtStat_Val_write/1
  Data Type Conversion12/1 -> IfVeSMSuStPassCmprtMd_Md10_CrtStat_Val_write/1
  Data Type Conversion13/1 -> IfVeSMSuStPassCmprtMd_Md11_CrtStat_Val_write/1
  Data Type Conversion14/1 -> IfVeSMSuStPassCmprtMd_Md12_CrtStat_Val_write/1
  Data Type Conversion15/1 -> IfVeSMSuStPassCmprtMd_Md13_CrtStat_Val_write/1
  Data Type Conversion16/1 -> IfVeSMSuStPassCmprtMd_Md14_CrtStat_Val_write/1
  Data Type Conversion17/1 -> IfVeSMSuStPassCmprtMd_Md15_CrtStat_Val_write/1
  Data Type Conversion18/1 -> IfVeSMSuStPassCmprtMd_Md16_CrtStat_Val_write/1
  Data Type Conversion19/1 -> IfVeSMSuStPassCmprtMd_Md17_CrtStat_Val_write/1
  Data Type Conversion20/1 -> IfVeSMSuStPassCmprtMd_Md18_CrtStat_Val_write/1
  Data Type Conversion21/1 -> IfVeSMSuStPassCmprtMd_Md19_CrtStat_Val_write/1
  Data Type Conversion22/1 -> IfVeSMSuStPassCmprtMd_Md2_CrtStat_Val_write/1
  Data Type Conversion23/1 -> IfVeSMSuStPassCmprtMd_Md20_CrtStat_Val_write/1
  Data Type Conversion24/1 -> IfVeSMSuStPassCmprtMd_Md21_CrtStat_Val_write/1
  Data Type Conversion25/1 -> IfVeSMSuStPassCmprtMd_Md22_CrtStat_Val_write/1
  Data Type Conversion26/1 -> IfVeSMSuStPassCmprtMd_Md23_CrtStat_Val_write/1
  Data Type Conversion27/1 -> IfVeSMSuStPassCmprtMd_Md24_CrtStat_Val_write/1
  Data Type Conversion28/1 -> IfVeSMSuStPassCmprtMd_Md25_CrtStat_Val_write/1
  Data Type Conversion29/1 -> IfVeSMSuStPassCmprtMd_Md26_CrtStat_Val_write/1
  Data Type Conversion30/1 -> IfVeSMSuStPassCmprtMd_Md27_CrtStat_Val_write/1
  Data Type Conversion31/1 -> IfVeSMSuStPassCmprtMd_Md28_CrtStat_Val_write/1
  Data Type Conversion32/1 -> IfVeSMSuStPassCmprtMd_Md29_CrtStat_Val_write/1
  Data Type Conversion33/1 -> IfVeSMSuStPassCmprtMd_Md3_CrtStat_Val_write/1
  Data Type Conversion34/1 -> IfVeSMSuStPassCmprtMd_Md30_CrtStat_Val_write/1
  Data Type Conversion35/1 -> IfVeSMSuStPassCmprtMd_Md31_CrtStat_Val_write/1
  Data Type Conversion36/1 -> IfVeSMSuStPassCmprtMd_Md32_CrtStat_Val_write/1
  Data Type Conversion37/1 -> IfVeSMSuStPassCmprtMd_Md4_CrtStat_Val_write/1
  Data Type Conversion38/1 -> IfVeSMSuStPassCmprtMd_Md5_CrtStat_Val_write/1
  Data Type Conversion39/1 -> IfVeSMSuStPassCmprtMd_Md6_CrtStat_Val_write/1
  Data Type Conversion40/1 -> IfVeSMSuStPassCmprtMd_Md7_CrtStat_Val_write/1
  Data Type Conversion41/1 -> IfVeSMSuStPassCmprtMd_Md8_CrtStat_Val_write/1
  Data Type Conversion42/1 -> IfVeSMSuStPassCmprtMd_Md9_CrtStat_Val_write/1
  Data Type Conversion43/1 -> IfVeSMSuStPassCmprtMdCrtMdStat_Val_write/1
  Data Type Conversion44/1 -> IfVeSMSuStPassCmprtMd_Md53_CrtStat_Val_write/1
  Data Type Conversion45/1 -> IfVeSMSuStPassCmprtMd_Md56_CrtStat_Val_write/1
  Subsystem/45(IfVeSMSuStPassCmprtMd_Md53_CrtStat_Val_write) -> Data Type Conversion44/1
  Subsystem/46(IfVeSMSuStPassCmprtMd_Md56_CrtStat_Val_write) -> Data Type Conversion45/1
  Data Type Conversion46/1 -> IfVeSMSuStPassCmprtMd_Md57_CrtStat_Val_write/1
  Data Type Conversion47/1 -> IfVeSMSuStPassCmprtMd_Md58_CrtStat_Val_write/1
  Subsystem/47(IfVeSMSuStPassCmprtMd_Md57_CrtStat_Val_write) -> Data Type Conversion46/1
  Subsystem/48(IfVeSMSuStPassCmprtMd_Md58_CrtStat_Val_write) -> Data Type Conversion47/1
  Data Type Conversion48/1 -> IfVeSMSuStPassCmprtMd_Md61_CrtStat_Val_write/1
  Data Type Conversion49/1 -> IfVeSMSuStPassCmprtMd_Md62_CrtStat_Val_write/1
  Subsystem/49(IfVeSMSuStPassCmprtMd_Md61_CrtStat_Val_write) -> Data Type Conversion48/1
  Subsystem/50(IfVeSMSuStPassCmprtMd_Md62_CrtStat_Val_write) -> Data Type Conversion49/1

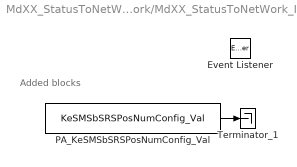
== system MdXX_StatusToNetWork/MdXX_StatusToNetWork_Init ==
  note: Added blocks
  Event Listener : EventListener  EventName=reset
  PA_KeSMSbSRSPosNumConfig_Val : Constant  Value=KeSMSbSRSPosNumConfig_Val
  Terminator_1 : Terminator
  wires:
  PA_KeSMSbSRSPosNumConfig_Val/1 -> Terminator_1/1
